simulink model "create_3D_animation"  (R2020a)
settings: Solver=VariableStepAuto  StartTime=0.0  StopTime=37  RelTol=1e-3
undefined symbols (not defined in the file): Psi, X, Y
libraries: sim3dautolib x5, sim3dlib x3, visionsinks x2, dspvision x1
settings Model: Creator=fvall  LastModifiedBy=fvall

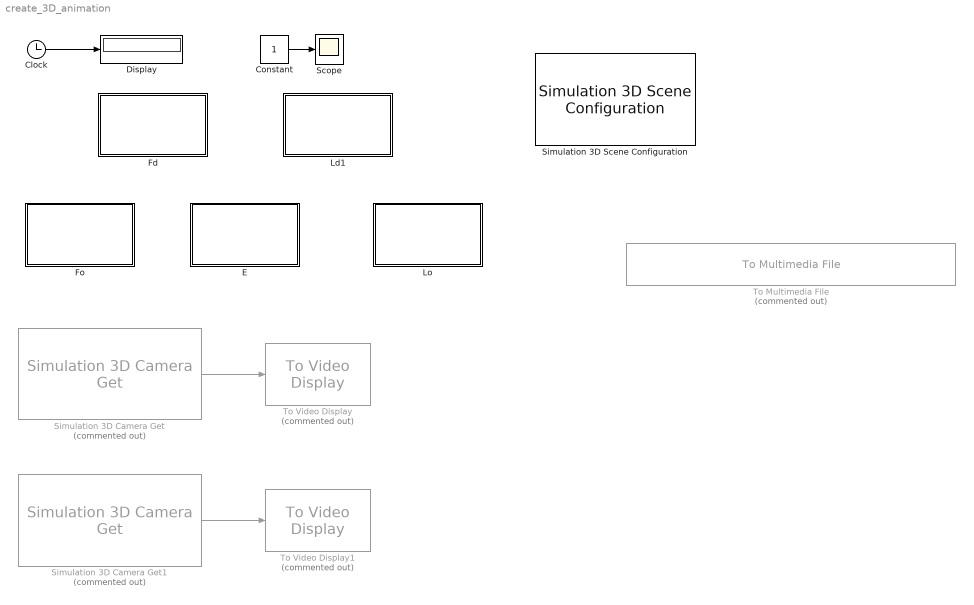
== system create_3D_animation ==
  Clock : Clock
  Constant : Constant
  Display : Display
  E : Subsystem  mask{ActorName=E, VehColor=Red, x=X{2}, y=Y{2}, psi=Psi{2}}
      mask prompts: ActorName "shared_sim3dblks:sim3dblkVehicleWithGroundFollowing:blkPrm_ActorName"; VehColor "shared_sim3dblks:sim3dblkVehicleWithGroundFollowing:blkPrm_VehColor"
      mask TypeOptions ActorName: Simulation 3D Vehicle with Ground Following/ActorName
      mask TypeOptions VehColor: Simulation 3D Vehicle with Ground Following/VehColor
      mask DialogControl vehParams Prompt: Vehicle Parameters
      mask DialogControl ActorName Prompt: Name:
      mask DialogControl VehColor Prompt: Color:
      mask DialogControl vehStates Prompt: Vehicle States
  Fd : Subsystem  mask{ActorName=Fd, VehColor=Green, x=X{5}, y=Y{5}, psi=Psi{5}}
      mask prompts: ActorName "shared_sim3dblks:sim3dblkVehicleWithGroundFollowing:blkPrm_ActorName"; VehColor "shared_sim3dblks:sim3dblkVehicleWithGroundFollowing:blkPrm_VehColor"
      mask TypeOptions ActorName: Simulation 3D Vehicle with Ground Following/ActorName
      mask TypeOptions VehColor: Simulation 3D Vehicle with Ground Following/VehColor
      mask DialogControl vehParams Prompt: Vehicle Parameters
      mask DialogControl ActorName Prompt: Name:
      mask DialogControl VehColor Prompt: Color:
      mask DialogControl vehStates Prompt: Vehicle States
  Fo : Subsystem  mask{ActorName=Fo, VehColor=Green, x=X{3}, y=Y{3}, psi=Psi{3}}
      mask prompts: ActorName "shared_sim3dblks:sim3dblkVehicleWithGroundFollowing:blkPrm_ActorName"; VehColor "shared_sim3dblks:sim3dblkVehicleWithGroundFollowing:blkPrm_VehColor"
      mask TypeOptions ActorName: Simulation 3D Vehicle with Ground Following/ActorName
      mask TypeOptions VehColor: Simulation 3D Vehicle with Ground Following/VehColor
      mask DialogControl vehParams Prompt: Vehicle Parameters
      mask DialogControl ActorName Prompt: Name:
      mask DialogControl VehColor Prompt: Color:
      mask DialogControl vehStates Prompt: Vehicle States
  Ld1 : Subsystem  mask{ActorName=Ld1, VehColor=Green, x=X{4}, y=Y{4}, psi=Psi{4}}
      mask prompts: ActorName "shared_sim3dblks:sim3dblkVehicleWithGroundFollowing:blkPrm_ActorName"; VehColor "shared_sim3dblks:sim3dblkVehicleWithGroundFollowing:blkPrm_VehColor"
      mask TypeOptions ActorName: Simulation 3D Vehicle with Ground Following/ActorName
      mask TypeOptions VehColor: Simulation 3D Vehicle with Ground Following/VehColor
      mask DialogControl vehParams Prompt: Vehicle Paramaters
      mask DialogControl ActorName Prompt: Name:
      mask DialogControl VehColor Prompt: Color:
      mask DialogControl vehStates Prompt: Vehicle States
  Lo : Subsystem  mask{ActorName=Lo, VehColor=Green, x=X{1}, y=Y{1}, psi=Psi{1}}
      mask prompts: ActorName "shared_sim3dblks:sim3dblkVehicleWithGroundFollowing:blkPrm_ActorName"; VehColor "shared_sim3dblks:sim3dblkVehicleWithGroundFollowing:blkPrm_VehColor"
      mask TypeOptions ActorName: Simulation 3D Vehicle with Ground Following/ActorName
      mask TypeOptions VehColor: Simulation 3D Vehicle with Ground Following/VehColor
      mask DialogControl vehParams Prompt: Vehicle Parameters
      mask DialogControl ActorName Prompt: Name:
      mask DialogControl VehColor Prompt: Color:
      mask DialogControl vehStates Prompt: Vehicle States
  Scope : Scope
  Simulation 3D Camera Get : sim3dlib/Simulation 3D Camera Get  Priority=1  Commented=on  sensorTag=Sim3dSensor1  sensorId=1  sensorName=Sim3dSensor1  vehTagList={'E';'Fd';'Fo';'Ld1';'Lo';'Scene Origin'}  vehTag=E  mountLoc=Rearview mirror  offsetFlag=off  tmountOffset=[0, 0, 0]  rmountOffset=[0, 0, 0]  HorizontalResolution=1280  VerticalResolution=720  HorizontalFOV=60  SampleTime=-1  mountPoint=[0.433999985456467 0 1.29999995231628]  mountOrientation=[0 0 0]  aMode=2  ID=1
      settings: SourceProductBaseCode=DR,VE
  Simulation 3D Camera Get1 : sim3dlib/Simulation 3D Camera Get  Priority=1  Commented=on  sensorTag=Sim3dSensor2  sensorId=2  sensorName=Sim3dSensor2  vehTagList={'E';'Fd';'Fo';'Ld1';'Lo';'Scene Origin'}  vehTag=Fd  mountLoc=Hood center  offsetFlag=off  tmountOffset=[0, 0, 0]  rmountOffset=[0, 0, 0]  HorizontalResolution=1280  VerticalResolution=720  HorizontalFOV=60  SampleTime=-1  mountPoint=[1.46399998664856 0 1.10000002384186]  mountOrientation=[0 0 0]  aMode=2  ID=2
      settings: SourceProductBaseCode=DR,VE
  Simulation 3D Scene Configuration : sim3dlib/Simulation 3D Scene Configuration  Priority=0  ProjectFormat=Default Scenes  SceneDesc=Straight road  ProjectName=VehicleSimulation.exe  ScenePath=/Game/Maps/HwStrght  vehTagList={'E';'Fd';'Fo';'Ld1';'Lo';'Scene Origin'}  vehTag=E  OpVisEn=off  Ts=1/60  EnableWindow=on  sensorTag=MainCamera1  sensorId=1  sensorName=MainCamera1  mountLoc=Origin  offsetFlag=off  tmountOffset=[0, 0, 0]  rmountOffset=[0, 0, 0]  HorizontalResolution=1280  VerticalResolution=720  HorizontalFOV=60  mountPoint=[0 0 0]  mountOrientation=[0 0 0]  aMode=3  ID=1
      settings: SourceProductBaseCode=DR,VE
  To Multimedia File : dspvision/To Multimedia File  Commented=on  outputFilename=.\videos\full_maneuver_single_veh_rel_vel_-5_with_comms_3D.avi  streamSelection=Video only  videoCompressor=MJPEG Compressor  audioCompressor=None (uncompressed)  imagePorts=One multidimensional signal  fileType=AVI  audioDatatype=Determine from input data type  fourcc=RGB  videoQuality=75  mj2000CompFactor=10
  To Video Display : visionsinks/To Video Display  Commented=on  windowSizeMode=Normal  openAtMdlStart=on  fullScreen=off  videoWindowX=536805376  videoWindowY=536805376  saveWindowSize=off  videoWindowWidth=2147483647  videoWindowHeight=2147483647  inputColorFormat=RGB  inputType=Obsolete  imagePorts=One multidimensional signal  OutputDevice=On-screen video monitor  dataOrg=Column-major  isWindowOpen=off
  To Video Display1 : visionsinks/To Video Display  Commented=on  windowSizeMode=Normal  openAtMdlStart=on  fullScreen=off  videoWindowX=536805376  videoWindowY=536805376  saveWindowSize=off  videoWindowWidth=2147483647  videoWindowHeight=2147483647  inputColorFormat=RGB  inputType=Obsolete  imagePorts=One multidimensional signal  OutputDevice=On-screen video monitor  dataOrg=Column-major  isWindowOpen=off
  wires:
  Simulation 3D Camera Get/1 -> To Video Display/1
  Clock/1 -> Display/1
  Constant/1 -> Scope/1
  Simulation 3D Camera Get1/1 -> To Video Display1/1

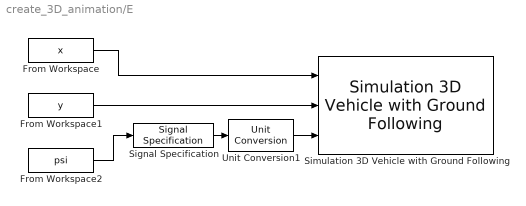
== system create_3D_animation/E ==
  From Workspace : FromWorkspace  VariableName=x
  From Workspace1 : FromWorkspace  VariableName=y
  From Workspace2 : FromWorkspace  VariableName=psi
  Signal Specification : SignalSpecification  Unit=rad
  Simulation 3D Vehicle with Ground Following : sim3dautolib/Simulation 3D Vehicle with Ground Following  Priority=-1  PassVehMesh=Sedan  VehColor=Red  InitialPos=[x.data(1), y.data(1), psi.data(1)]  InitialRot=[0, 0, 0]  ActorName=E  SampleTime=-1  ActorType=SimulinkVehicle  ID=C  aMode=3  ActorTag=E  CoordinateScheme=ISO  TransformOutportEnabled=off
      settings: SourceProductBaseCode=DR,VE
  Unit Conversion1 : UnitConversion
  wires:
  From Workspace/1 -> Simulation 3D Vehicle with Ground Following/1
  Signal Specification/1 -> Unit Conversion1/1
  Unit Conversion1/1 -> Simulation 3D Vehicle with Ground Following/3
  From Workspace1/1 -> Simulation 3D Vehicle with Ground Following/2
  From Workspace2/1 -> Signal Specification/1

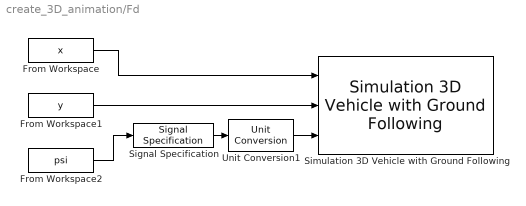
== system create_3D_animation/Fd ==
  From Workspace : FromWorkspace  VariableName=x
  From Workspace1 : FromWorkspace  VariableName=y
  From Workspace2 : FromWorkspace  VariableName=psi
  Signal Specification : SignalSpecification  Unit=rad
  Simulation 3D Vehicle with Ground Following : sim3dautolib/Simulation 3D Vehicle with Ground Following  Priority=-1  PassVehMesh=Sedan  VehColor=Green  InitialPos=[x.data(1), y.data(1), psi.data(1)]  InitialRot=[0, 0, 0]  ActorName=Fd  SampleTime=-1  ActorType=SimulinkVehicle  ID=C  aMode=3  ActorTag=Fd  CoordinateScheme=ISO  TransformOutportEnabled=off
      settings: SourceProductBaseCode=DR,VE
  Unit Conversion1 : UnitConversion
  wires:
  From Workspace2/1 -> Signal Specification/1
  From Workspace1/1 -> Simulation 3D Vehicle with Ground Following/2
  Unit Conversion1/1 -> Simulation 3D Vehicle with Ground Following/3
  Signal Specification/1 -> Unit Conversion1/1
  From Workspace/1 -> Simulation 3D Vehicle with Ground Following/1

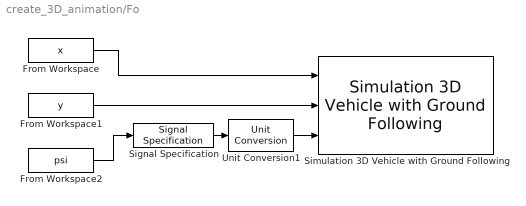
== system create_3D_animation/Fo ==
  From Workspace : FromWorkspace  VariableName=x
  From Workspace1 : FromWorkspace  VariableName=y
  From Workspace2 : FromWorkspace  VariableName=psi
  Signal Specification : SignalSpecification  Unit=rad
  Simulation 3D Vehicle with Ground Following : sim3dautolib/Simulation 3D Vehicle with Ground Following  Priority=-1  PassVehMesh=Sedan  VehColor=Green  InitialPos=[x.data(1), y.data(1), psi.data(1)]  InitialRot=[0, 0, 0]  ActorName=Fo  SampleTime=-1  ActorType=SimulinkVehicle  ID=C  aMode=3  ActorTag=Fo  CoordinateScheme=ISO  TransformOutportEnabled=off
      settings: SourceProductBaseCode=DR,VE
  Unit Conversion1 : UnitConversion
  wires:
  From Workspace2/1 -> Signal Specification/1
  From Workspace1/1 -> Simulation 3D Vehicle with Ground Following/2
  Unit Conversion1/1 -> Simulation 3D Vehicle with Ground Following/3
  Signal Specification/1 -> Unit Conversion1/1
  From Workspace/1 -> Simulation 3D Vehicle with Ground Following/1

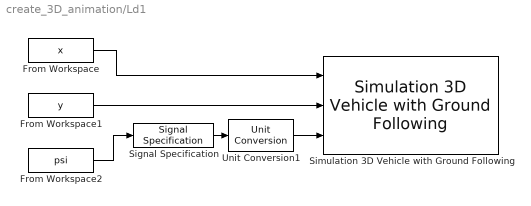
== system create_3D_animation/Ld1 ==
  From Workspace : FromWorkspace  VariableName=x
  From Workspace1 : FromWorkspace  VariableName=y
  From Workspace2 : FromWorkspace  VariableName=psi
  Signal Specification : SignalSpecification  Unit=rad
  Simulation 3D Vehicle with Ground Following : sim3dautolib/Simulation 3D Vehicle with Ground Following  Priority=-1  PassVehMesh=Sedan  VehColor=Green  InitialPos=[x.data(1), y.data(1), psi.data(1)]  InitialRot=[0, 0, 0]  ActorName=Ld1  SampleTime=-1  ActorType=SimulinkVehicle  ID=C  aMode=3  ActorTag=Ld1  CoordinateScheme=ISO  TransformOutportEnabled=off
      settings: SourceProductBaseCode=DR,VE
  Unit Conversion1 : UnitConversion
  wires:
  From Workspace2/1 -> Signal Specification/1
  Signal Specification/1 -> Unit Conversion1/1
  Unit Conversion1/1 -> Simulation 3D Vehicle with Ground Following/3
  From Workspace1/1 -> Simulation 3D Vehicle with Ground Following/2
  From Workspace/1 -> Simulation 3D Vehicle with Ground Following/1

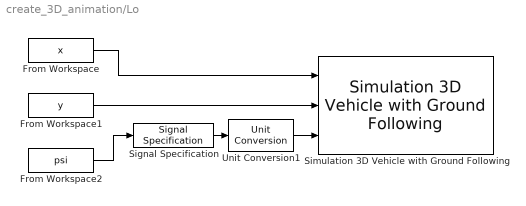
== system create_3D_animation/Lo ==
  From Workspace : FromWorkspace  VariableName=x
  From Workspace1 : FromWorkspace  VariableName=y
  From Workspace2 : FromWorkspace  VariableName=psi
  Signal Specification : SignalSpecification  Unit=rad
  Simulation 3D Vehicle with Ground Following : sim3dautolib/Simulation 3D Vehicle with Ground Following  Priority=-1  PassVehMesh=Sedan  VehColor=Green  InitialPos=[x.data(1), y.data(1), psi.data(1)]  InitialRot=[0, 0, 0]  ActorName=Lo  SampleTime=-1  ActorType=SimulinkVehicle  ID=C  aMode=3  ActorTag=Lo  CoordinateScheme=ISO  TransformOutportEnabled=off
      settings: SourceProductBaseCode=DR,VE
  Unit Conversion1 : UnitConversion
  wires:
  From Workspace/1 -> Simulation 3D Vehicle with Ground Following/1
  Signal Specification/1 -> Unit Conversion1/1
  Unit Conversion1/1 -> Simulation 3D Vehicle with Ground Following/3
  From Workspace1/1 -> Simulation 3D Vehicle with Ground Following/2
  From Workspace2/1 -> Signal Specification/1
